simulink library "CrazyFlie_lib"  (R2015a)
settings: Solver=ode45  StartTime=0.0  StopTime=10.0  RelTol=1e-3
settings Model: Creator=rshum  LastModifiedBy=rshum

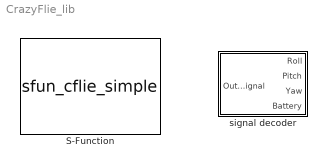
== system CrazyFlie_lib ==
  S-Function : S-Function  FunctionName=sfun_cflie_simple  Parameters=1
      mask Display: image(imread('crazyflie.jpg'))
  signal decoder : Subsystem

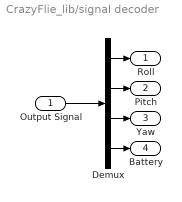
== system CrazyFlie_lib/signal decoder ==
  Output Signal : Inport
  Demux : Demux
  Roll : Outport
  Pitch : Outport  Port=2
  Yaw : Outport  Port=3
  Battery : Outport  Port=4
  wires:
  Demux/1 -> Roll/1
  Demux/3 -> Yaw/1
  Demux/2 -> Pitch/1
  Demux/4 -> Battery/1
  Output Signal/1 -> Demux/1
